simulink model "Quintic_Controller_max_distance"  (R2021a)
settings: Solver=VariableStepAuto  StartTime=0.0  StopTime=1.5  FixedStep=0.00005  MaxStep=.01  RelTol=1e-4  AbsTol=1e-4
values from neighbouring files (symbols this model uses):
  Angle_noise = 0.000001    (= 1e-06)    [Parameters.m]
  Current_noise = 0.000001    (= 1e-06)    [Parameters.m]
  F_sampling = 128    [Parameters.m]
  J_load = J_arm + (J_ball + m_ball*r_arm^2) + J_rotor    (= 0.00716067135)    [Parameters.m]
  J_rotor = 0.0000795    (= 7.95e-05)    [Parameters.m]
  kd_q = 400    [Parameters.m]
  ki_c = 100    [Parameters.m]
  ki_q = 0.01    [Parameters.m]
  ki_s = 4    [Parameters.m]
  km = kt/sqrt(Rm)    [Parameters.m]
  kp_c = 23    [Parameters.m]
  kp_q = 10    [Parameters.m]
  kp_s = 10    [Parameters.m]
  n = 3.75    [Parameters.m]
  nu = 0.85    [Parameters.m]
  Velocity_noise = 0.000001    (= 1e-06)    [Parameters.m]
  x0 = -0.45697770542    [Parameters.m]    (also in getBallPos.m)
  y0 = -0.02848783783    [Parameters.m]    (also in getBallPos.m)
undefined symbols (not defined in the file or in its folder): smiData, X, Y, Z
libraries: sm_lib x103, nesl_utility x12, fl_lib x9, simulink x6, ee_lib x4, spsSampleandHoldLib x3, pid_lib x2, sdl_lib x1
(part 3 of 3)

== system Quintic_Controller_max_distance/Motor ==
  ReferenceFrame : sm_lib/Frames and Transforms/Reference Frame
  Solid : sm_lib/Body Elements/File Solid  ExtGeomFileName=Motor_Default_sldprt.STEP  UnitType=FromFile  ExtGeomFileUnits=m  StepReaderType=HEX  ExportConvexHullGeometry=off  InertiaType=Custom  Mass=smiData.Solid(5).mass  MassUnits=kg  CenterOfMass=smiData.Solid(5).CoM  CenterOfMassUnits=mm  MomentsOfInertia=smiData.Solid(5).MoI  MomentsOfInertiaUnits=kg*mm^2  ProductsOfInertia=smiData.Solid(5).PoI  ProductsOfInertiaUnits=kg*mm^2  BasedOnType=DensityFromFile  Density=1000  DensityUnits=kg/m^3  DoExposeReferenceFrame=on  SerializedFrames=<Frames/>  GraphicType=FromGeometry  MarkerShape=Sphere  MarkerSize=10  GraphicVisPropType=SimpleVisualProperties  GraphicDiffuseColor=smiData.Solid(5).color  GraphicSpecularColor=[0.5 0.5 0.5 1.0]  GraphicAmbientColor=[0.15 0.15 0.15 1.0]  GraphicEmissiveColor=[0.0 0.0 0.0 1.0]  GraphicShininess=75  GraphicOpacity=smiData.Solid(5).opacity
  Transform : sm_lib/Frames and Transforms/Rigid Transform  TranslationMethod=Cartesian  TranslationStandardOffset=0  TranslationLengthUnit=mm  TranslationStandardAxis=+Z  TranslationCartesianOffset=smiData.RigidTransform(28).translation  TranslationROffset=0  TranslationROffsetUnits=m  TranslationZOffset=0  TranslationZOffsetUnits=m  TranslationThetaOffset=0  TranslationThetaOffsetUnits=deg  RotationMethod=ArbitraryAxis  RotationAngleUnits=rad  RotationStandardAxis=+Z  RotationAngle=smiData.RigidTransform(28).angle  RotationArbitraryAxis=smiData.RigidTransform(28).axis  FollAlignAxisA=+X  BaseAlignAxisA=+Y  FollAlignAxisB=+Y  BaseAlignAxisB=+Z  RotationSequenceAxes=FollowerAxes  RotationSequence=XYX  RotationSequenceAngles=[0 0 0]  RotationSequenceAnglesUnits=deg  RotationMatrix=[1 0 0; 0 1 0; 0 0 1]
  Transform1 : sm_lib/Frames and Transforms/Rigid Transform  TranslationMethod=Cartesian  TranslationStandardOffset=0  TranslationLengthUnit=mm  TranslationStandardAxis=+Z  TranslationCartesianOffset=smiData.RigidTransform(45).translation  TranslationROffset=0  TranslationROffsetUnits=m  TranslationZOffset=0  TranslationZOffsetUnits=m  TranslationThetaOffset=0  TranslationThetaOffsetUnits=deg  RotationMethod=ArbitraryAxis  RotationAngleUnits=rad  RotationStandardAxis=+Z  RotationAngle=smiData.RigidTransform(45).angle  RotationArbitraryAxis=smiData.RigidTransform(45).axis  FollAlignAxisA=+X  BaseAlignAxisA=+Y  FollAlignAxisB=+Y  BaseAlignAxisB=+Z  RotationSequenceAxes=FollowerAxes  RotationSequence=XYX  RotationSequenceAngles=[0 0 0]  RotationSequenceAnglesUnits=deg  RotationMatrix=[1 0 0; 0 1 0; 0 0 1]
  F : PMIOPort  Side=Left
  F1 : PMIOPort  Port=2  Side=Right
  connections:
  ReferenceFrame/RConn1 -- Solid/RConn1 -- Transform/LConn1 -- Transform1/LConn1
  Transform/RConn1 -- F/RConn1
  Transform1/RConn1 -- F1/RConn1

== system Quintic_Controller_max_distance/Motor Mount ==
  ReferenceFrame : sm_lib/Frames and Transforms/Reference Frame
  Solid : sm_lib/Body Elements/File Solid  ExtGeomFileName=8982K141_Multipurpose 6061 Aluminum 90 Degree Angle_8982K141_sldprt.STEP  UnitType=FromFile  ExtGeomFileUnits=m  StepReaderType=HEX  ExportConvexHullGeometry=off  InertiaType=Custom  Mass=smiData.Solid(4).mass  MassUnits=kg  CenterOfMass=smiData.Solid(4).CoM  CenterOfMassUnits=in  MomentsOfInertia=smiData.Solid(4).MoI  MomentsOfInertiaUnits=kg*in^2  ProductsOfInertia=smiData.Solid(4).PoI  ProductsOfInertiaUnits=kg*in^2  BasedOnType=DensityFromFile  Density=1000  DensityUnits=kg/m^3  DoExposeReferenceFrame=on  SerializedFrames=<Frames/>  GraphicType=FromGeometry  MarkerShape=Sphere  MarkerSize=10  GraphicVisPropType=SimpleVisualProperties  GraphicDiffuseColor=smiData.Solid(4).color  GraphicSpecularColor=[0.5 0.5 0.5 1.0]  GraphicAmbientColor=[0.15 0.15 0.15 1.0]  GraphicEmissiveColor=[0.0 0.0 0.0 1.0]  GraphicShininess=75  GraphicOpacity=smiData.Solid(4).opacity
  Transform : sm_lib/Frames and Transforms/Rigid Transform  TranslationMethod=Cartesian  TranslationStandardOffset=0  TranslationLengthUnit=mm  TranslationStandardAxis=+Z  TranslationCartesianOffset=smiData.RigidTransform(26).translation  TranslationROffset=0  TranslationROffsetUnits=m  TranslationZOffset=0  TranslationZOffsetUnits=m  TranslationThetaOffset=0  TranslationThetaOffsetUnits=deg  RotationMethod=ArbitraryAxis  RotationAngleUnits=rad  RotationStandardAxis=+Z  RotationAngle=smiData.RigidTransform(26).angle  RotationArbitraryAxis=smiData.RigidTransform(26).axis  FollAlignAxisA=+X  BaseAlignAxisA=+Y  FollAlignAxisB=+Y  BaseAlignAxisB=+Z  RotationSequenceAxes=FollowerAxes  RotationSequence=XYX  RotationSequenceAngles=[0 0 0]  RotationSequenceAnglesUnits=deg  RotationMatrix=[1 0 0; 0 1 0; 0 0 1]
  Transform1 : sm_lib/Frames and Transforms/Rigid Transform  TranslationMethod=Cartesian  TranslationStandardOffset=0  TranslationLengthUnit=mm  TranslationStandardAxis=+Z  TranslationCartesianOffset=smiData.RigidTransform(27).translation  TranslationROffset=0  TranslationROffsetUnits=m  TranslationZOffset=0  TranslationZOffsetUnits=m  TranslationThetaOffset=0  TranslationThetaOffsetUnits=deg  RotationMethod=ArbitraryAxis  RotationAngleUnits=rad  RotationStandardAxis=+Z  RotationAngle=smiData.RigidTransform(27).angle  RotationArbitraryAxis=smiData.RigidTransform(27).axis  FollAlignAxisA=+X  BaseAlignAxisA=+Y  FollAlignAxisB=+Y  BaseAlignAxisB=+Z  RotationSequenceAxes=FollowerAxes  RotationSequence=XYX  RotationSequenceAngles=[0 0 0]  RotationSequenceAnglesUnits=deg  RotationMatrix=[1 0 0; 0 1 0; 0 0 1]
  Transform2 : sm_lib/Frames and Transforms/Rigid Transform  TranslationMethod=Cartesian  TranslationStandardOffset=0  TranslationLengthUnit=mm  TranslationStandardAxis=+Z  TranslationCartesianOffset=smiData.RigidTransform(44).translation  TranslationROffset=0  TranslationROffsetUnits=m  TranslationZOffset=0  TranslationZOffsetUnits=m  TranslationThetaOffset=0  TranslationThetaOffsetUnits=deg  RotationMethod=ArbitraryAxis  RotationAngleUnits=rad  RotationStandardAxis=+Z  RotationAngle=smiData.RigidTransform(44).angle  RotationArbitraryAxis=smiData.RigidTransform(44).axis  FollAlignAxisA=+X  BaseAlignAxisA=+Y  FollAlignAxisB=+Y  BaseAlignAxisB=+Z  RotationSequenceAxes=FollowerAxes  RotationSequence=XYX  RotationSequenceAngles=[0 0 0]  RotationSequenceAnglesUnits=deg  RotationMatrix=[1 0 0; 0 1 0; 0 0 1]
  F1 : PMIOPort  Side=Left
  F2 : PMIOPort  Port=2  Side=Left
  F : PMIOPort  Port=3  Side=Left
  connections:
  ReferenceFrame/RConn1 -- Solid/RConn1 -- Transform/LConn1 -- Transform1/LConn1 -- Transform2/LConn1
  Transform/RConn1 -- F/RConn1
  Transform1/RConn1 -- F1/RConn1
  Transform2/RConn1 -- F2/RConn1

== system Quintic_Controller_max_distance/Output Gear ==
  ReferenceFrame : sm_lib/Frames and Transforms/Reference Frame
  Solid : sm_lib/Body Elements/File Solid  ExtGeomFileName=2664N150_METAL GEAR - 20 DEGREE PRESSURE ANGLE_2664N15_sldprt.STEP  UnitType=FromFile  ExtGeomFileUnits=m  StepReaderType=HEX  ExportConvexHullGeometry=off  InertiaType=Custom  Mass=smiData.Solid(7).mass  MassUnits=kg  CenterOfMass=smiData.Solid(7).CoM  CenterOfMassUnits=in  MomentsOfInertia=smiData.Solid(7).MoI  MomentsOfInertiaUnits=kg*in^2  ProductsOfInertia=smiData.Solid(7).PoI  ProductsOfInertiaUnits=kg*in^2  BasedOnType=DensityFromFile  Density=1000  DensityUnits=kg/m^3  DoExposeReferenceFrame=on  SerializedFrames=<Frames/>  GraphicType=FromGeometry  MarkerShape=Sphere  MarkerSize=10  GraphicVisPropType=SimpleVisualProperties  GraphicDiffuseColor=smiData.Solid(7).color  GraphicSpecularColor=[0.5 0.5 0.5 1.0]  GraphicAmbientColor=[0.15 0.15 0.15 1.0]  GraphicEmissiveColor=[0.0 0.0 0.0 1.0]  GraphicShininess=75  GraphicOpacity=smiData.Solid(7).opacity
  Transform : sm_lib/Frames and Transforms/Rigid Transform  TranslationMethod=Cartesian  TranslationStandardOffset=0  TranslationLengthUnit=mm  TranslationStandardAxis=+Z  TranslationCartesianOffset=smiData.RigidTransform(40).translation  TranslationROffset=0  TranslationROffsetUnits=m  TranslationZOffset=0  TranslationZOffsetUnits=m  TranslationThetaOffset=0  TranslationThetaOffsetUnits=deg  RotationMethod=ArbitraryAxis  RotationAngleUnits=rad  RotationStandardAxis=+Z  RotationAngle=smiData.RigidTransform(40).angle  RotationArbitraryAxis=smiData.RigidTransform(40).axis  FollAlignAxisA=+X  BaseAlignAxisA=+Y  FollAlignAxisB=+Y  BaseAlignAxisB=+Z  RotationSequenceAxes=FollowerAxes  RotationSequence=XYX  RotationSequenceAngles=[0 0 0]  RotationSequenceAnglesUnits=deg  RotationMatrix=[1 0 0; 0 1 0; 0 0 1]
  Transform1 : sm_lib/Frames and Transforms/Rigid Transform  TranslationMethod=Cartesian  TranslationStandardOffset=0  TranslationLengthUnit=mm  TranslationStandardAxis=+Z  TranslationCartesianOffset=smiData.RigidTransform(41).translation  TranslationROffset=0  TranslationROffsetUnits=m  TranslationZOffset=0  TranslationZOffsetUnits=m  TranslationThetaOffset=0  TranslationThetaOffsetUnits=deg  RotationMethod=ArbitraryAxis  RotationAngleUnits=rad  RotationStandardAxis=+Z  RotationAngle=smiData.RigidTransform(41).angle  RotationArbitraryAxis=smiData.RigidTransform(41).axis  FollAlignAxisA=+X  BaseAlignAxisA=+Y  FollAlignAxisB=+Y  BaseAlignAxisB=+Z  RotationSequenceAxes=FollowerAxes  RotationSequence=XYX  RotationSequenceAngles=[0 0 0]  RotationSequenceAnglesUnits=deg  RotationMatrix=[1 0 0; 0 1 0; 0 0 1]
  F : PMIOPort  Side=Left
  F1 : PMIOPort  Port=2  Side=Right
  connections:
  ReferenceFrame/RConn1 -- Solid/RConn1 -- Transform/LConn1 -- Transform1/LConn1
  Transform/RConn1 -- F/RConn1
  Transform1/RConn1 -- F1/RConn1

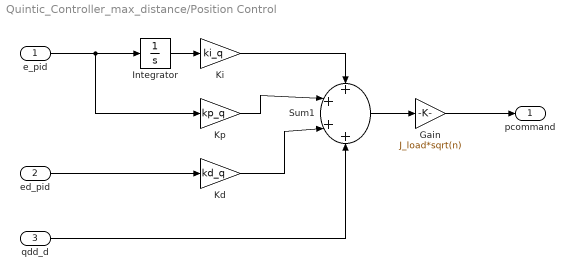
== system Quintic_Controller_max_distance/Position Control ==
  e_pid : Inport
  ed_pid : Inport  Port=2
  qdd_d : Inport  Port=3
  Gain : Gain  Gain=J_load*sqrt(n)
  Integrator : Integrator
  Kd : Gain  Gain=kd_q
  Ki : Gain  Gain=ki_q
  Kp : Gain  Gain=kp_q
  Sum1 : Sum  Inputs=++++
  pcommand : Outport
  wires:
  e_pid/1 -> Integrator/1, Kp/1
  ed_pid/1 -> Kd/1
  Integrator/1 -> Ki/1
  Kp/1 -> Sum1/2
  Sum1/1 -> Gain/1
  Ki/1 -> Sum1/1
  Kd/1 -> Sum1/3
  qdd_d/1 -> Sum1/4
  Gain/1 -> pcommand/1

== system Quintic_Controller_max_distance/Power Sens ==
  Integrator : Integrator
  PS-Simulink Converter8 : nesl_utility/PS-Simulink Converter  PhysicalDomain=network_engine_domain  SubClassName=ps_output  LeftPortType=input  RightPortType=output  PseudoPeriodic=off  Frequencies=[]  Unit=inherit  AffineConversion=off
      settings: SourceProductBaseCode=PW,SS
  Power : Scope
  Power Sensor : ee_lib/Sensors & Transducers/Power Sensor  measurement_type=1  averaging_period=1e-4 s
      settings: SourceProductBaseCode=PS
  To Workspace : ToWorkspace  VariableName=total_power  SaveFormat=Timeseries  SampleTime=-1
  Source : PMIOPort  Side=Left
  + : PMIOPort  Port=2  Side=Left
  GND : PMIOPort  Port=3  Side=Left
  wires:
  PS-Simulink Converter8/1 -> Integrator/1
  Integrator/1 -> To Workspace/1, Power/1
  connections:
  Power Sensor/LConn3 -- GND/RConn1
  Power Sensor/RConn1 -- PS-Simulink Converter8/LConn1
  Power Sensor/LConn2 -- +/RConn1
  Power Sensor/LConn1 -- Source/RConn1

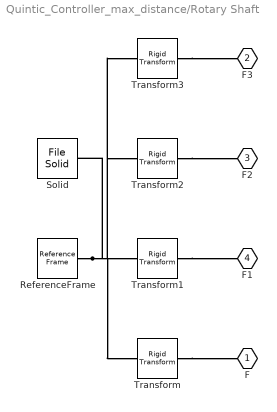
== system Quintic_Controller_max_distance/Rotary Shaft ==
  ReferenceFrame : sm_lib/Frames and Transforms/Reference Frame
  Solid : sm_lib/Body Elements/File Solid  ExtGeomFileName=1439K411_1045 Carbon Steel Keyed Rotary Shaft_1439K411_sldprt.STEP  UnitType=FromFile  ExtGeomFileUnits=m  StepReaderType=HEX  ExportConvexHullGeometry=off  InertiaType=Custom  Mass=smiData.Solid(10).mass  MassUnits=kg  CenterOfMass=smiData.Solid(10).CoM  CenterOfMassUnits=mm  MomentsOfInertia=smiData.Solid(10).MoI  MomentsOfInertiaUnits=kg*mm^2  ProductsOfInertia=smiData.Solid(10).PoI  ProductsOfInertiaUnits=kg*mm^2  BasedOnType=DensityFromFile  Density=1000  DensityUnits=kg/m^3  DoExposeReferenceFrame=on  SerializedFrames=<Frames/>  GraphicType=FromGeometry  MarkerShape=Sphere  MarkerSize=10  GraphicVisPropType=SimpleVisualProperties  GraphicDiffuseColor=smiData.Solid(10).color  GraphicSpecularColor=[0.5 0.5 0.5 1.0]  GraphicAmbientColor=[0.15 0.15 0.15 1.0]  GraphicEmissiveColor=[0.0 0.0 0.0 1.0]  GraphicShininess=75  GraphicOpacity=smiData.Solid(10).opacity
  Transform : sm_lib/Frames and Transforms/Rigid Transform  TranslationMethod=Cartesian  TranslationStandardOffset=0  TranslationLengthUnit=mm  TranslationStandardAxis=+Z  TranslationCartesianOffset=smiData.RigidTransform(24).translation  TranslationROffset=0  TranslationROffsetUnits=m  TranslationZOffset=0  TranslationZOffsetUnits=m  TranslationThetaOffset=0  TranslationThetaOffsetUnits=deg  RotationMethod=ArbitraryAxis  RotationAngleUnits=rad  RotationStandardAxis=+Z  RotationAngle=smiData.RigidTransform(24).angle  RotationArbitraryAxis=smiData.RigidTransform(24).axis  FollAlignAxisA=+X  BaseAlignAxisA=+Y  FollAlignAxisB=+Y  BaseAlignAxisB=+Z  RotationSequenceAxes=FollowerAxes  RotationSequence=XYX  RotationSequenceAngles=[0 0 0]  RotationSequenceAnglesUnits=deg  RotationMatrix=[1 0 0; 0 1 0; 0 0 1]
  Transform1 : sm_lib/Frames and Transforms/Rigid Transform  TranslationMethod=Cartesian  TranslationStandardOffset=0  TranslationLengthUnit=mm  TranslationStandardAxis=+Z  TranslationCartesianOffset=smiData.RigidTransform(29).translation  TranslationROffset=0  TranslationROffsetUnits=m  TranslationZOffset=0  TranslationZOffsetUnits=m  TranslationThetaOffset=0  TranslationThetaOffsetUnits=deg  RotationMethod=ArbitraryAxis  RotationAngleUnits=rad  RotationStandardAxis=+Z  RotationAngle=smiData.RigidTransform(29).angle  RotationArbitraryAxis=smiData.RigidTransform(29).axis  FollAlignAxisA=+X  BaseAlignAxisA=+Y  FollAlignAxisB=+Y  BaseAlignAxisB=+Z  RotationSequenceAxes=FollowerAxes  RotationSequence=XYX  RotationSequenceAngles=[0 0 0]  RotationSequenceAnglesUnits=deg  RotationMatrix=[1 0 0; 0 1 0; 0 0 1]
  Transform2 : sm_lib/Frames and Transforms/Rigid Transform  TranslationMethod=Cartesian  TranslationStandardOffset=0  TranslationLengthUnit=mm  TranslationStandardAxis=+Z  TranslationCartesianOffset=smiData.RigidTransform(37).translation  TranslationROffset=0  TranslationROffsetUnits=m  TranslationZOffset=0  TranslationZOffsetUnits=m  TranslationThetaOffset=0  TranslationThetaOffsetUnits=deg  RotationMethod=ArbitraryAxis  RotationAngleUnits=rad  RotationStandardAxis=+Z  RotationAngle=smiData.RigidTransform(37).angle  RotationArbitraryAxis=smiData.RigidTransform(37).axis  FollAlignAxisA=+X  BaseAlignAxisA=+Y  FollAlignAxisB=+Y  BaseAlignAxisB=+Z  RotationSequenceAxes=FollowerAxes  RotationSequence=XYX  RotationSequenceAngles=[0 0 0]  RotationSequenceAnglesUnits=deg  RotationMatrix=[1 0 0; 0 1 0; 0 0 1]
  Transform3 : sm_lib/Frames and Transforms/Rigid Transform  TranslationMethod=Cartesian  TranslationStandardOffset=0  TranslationLengthUnit=mm  TranslationStandardAxis=+Z  TranslationCartesianOffset=smiData.RigidTransform(39).translation  TranslationROffset=0  TranslationROffsetUnits=m  TranslationZOffset=0  TranslationZOffsetUnits=m  TranslationThetaOffset=0  TranslationThetaOffsetUnits=deg  RotationMethod=ArbitraryAxis  RotationAngleUnits=rad  RotationStandardAxis=+Z  RotationAngle=smiData.RigidTransform(39).angle  RotationArbitraryAxis=smiData.RigidTransform(39).axis  FollAlignAxisA=+X  BaseAlignAxisA=+Y  FollAlignAxisB=+Y  BaseAlignAxisB=+Z  RotationSequenceAxes=FollowerAxes  RotationSequence=XYX  RotationSequenceAngles=[0 0 0]  RotationSequenceAnglesUnits=deg  RotationMatrix=[1 0 0; 0 1 0; 0 0 1]
  F : PMIOPort  Side=Left
  F3 : PMIOPort  Port=2  Side=Right
  F2 : PMIOPort  Port=3  Side=Right
  F1 : PMIOPort  Port=4  Side=Right
  connections:
  ReferenceFrame/RConn1 -- Solid/RConn1 -- Transform/LConn1 -- Transform1/LConn1 -- Transform2/LConn1 -- Transform3/LConn1
  Transform/RConn1 -- F/RConn1
  Transform1/RConn1 -- F1/RConn1
  Transform2/RConn1 -- F2/RConn1
  Transform3/RConn1 -- F3/RConn1

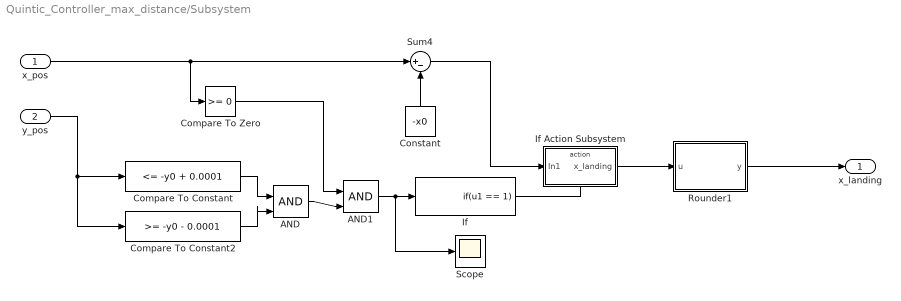
== system Quintic_Controller_max_distance/Subsystem ==
  x_pos : Inport
  y_pos : Inport  Port=2
  AND : Logic  IconShape=distinctive  AllPortsSameDT=off  OutDataTypeStr=boolean
  AND1 : Logic  IconShape=distinctive  AllPortsSameDT=off  OutDataTypeStr=boolean
  Compare To Constant : simulink/Logic and Bit Operations/Compare To Constant  relop=<=  const=-y0 + 0.0001  OutDataTypeStr=boolean
  Compare To Constant2 : simulink/Logic and Bit Operations/Compare To Constant  relop=>=  const=-y0 - 0.0001  OutDataTypeStr=boolean
  Compare To Zero : simulink/Logic and Bit Operations/Compare To Zero  relop=>=  OutDataTypeStr=boolean
  Constant : Constant  Value=-x0
  If : If  IfExpression=u1 == 1  ShowElse=off
  If Action Subsystem : Subsystem  TreatAsAtomicUnit=on
  Rounder1 : MATLAB Function  TreatAsAtomicUnit=on
  Scope : Scope
  Sum4 : Sum  Inputs=|+-
  x_landing : Outport
  wires:
  AND/1 -> AND1/2
  Compare To Constant2/1 -> AND/2
  y_pos/1 -> Compare To Constant2/1, Compare To Constant/1
  If/1 -> If Action Subsystem/Action
  Compare To Constant/1 -> AND/1
  Compare To Zero/1 -> AND1/1
  AND1/1 -> Scope/1, If/1
  Sum4/1 -> If Action Subsystem/1(In1)
  x_pos/1 -> Sum4/1, Compare To Zero/1
  Constant/1 -> Sum4/2
  If Action Subsystem/1(x_landing) -> Rounder1/1(u)
  Rounder1/1(y) -> x_landing/1

== system Quintic_Controller_max_distance/Velocity Sample//Noise Selector ==
  In1 : Inport
  Noise3 : Subsystem
  Sample3 : Subsystem  Commented=through
  Switch1 : Switch  Criteria=u2 > Threshold
  Switch2 : Switch  Criteria=u2 > Threshold
  Velocity Noise : Constant  Value=0
  Velocity Sample : Constant  Value=0
  Out1 : Outport
  wires:
  Switch1/1 -> Switch2/3, Sample3/1(In1)
  Sample3/1("   ") -> Switch2/1
  Velocity Noise/1 -> Switch1/2
  Switch2/1 -> Out1/1
  In1/1 -> Noise3/1(In1), Switch1/3
  Noise3/1(Out1) -> Switch1/1
  Velocity Sample/1 -> Switch2/2

== system Quintic_Controller_max_distance/Angle Sample//Noise Selector1/Noise3 ==
  In1 : Inport
  Band-Limited White Noise : simulink/Sources/Band-Limited White Noise  Cov=[Angle_noise]  Ts=0.001  seed=[23341]
  Sum3 : Sum  Inputs=|++
  Out1 : Outport
  wires:
  Band-Limited White Noise/1 -> Sum3/1
  In1/1 -> Sum3/2
  Sum3/1 -> Out1/1

== system Quintic_Controller_max_distance/Angle Sample//Noise Selector1/Sample3 ==
  In1 : Inport
  Pulse Generator : DiscretePulseGenerator  PulseType=Time based  Period=1/F_sampling
  Sample and Hold : spsSampleandHoldLib/Sample and Hold  ic=0  Ts=0
      settings: SourceProductBaseCode=PS
  "   " : Outport
  wires:
  Pulse Generator/1 -> Sample and Hold/2
  Sample and Hold/1 -> "   "/1
  In1/1 -> Sample and Hold/1

== system Quintic_Controller_max_distance/Current Sample//Noise Selector/Noise3 ==
  In1 : Inport
  Band-Limited White Noise : simulink/Sources/Band-Limited White Noise  Cov=[Current_noise]  Ts=0.001  seed=[23341]
  Sum3 : Sum  Inputs=|++
  Out1 : Outport
  wires:
  Band-Limited White Noise/1 -> Sum3/1
  In1/1 -> Sum3/2
  Sum3/1 -> Out1/1

== system Quintic_Controller_max_distance/Current Sample//Noise Selector/Sample3 ==
  In1 : Inport
  Pulse Generator : DiscretePulseGenerator  PulseType=Time based  Period=1/F_sampling
  Sample and Hold : spsSampleandHoldLib/Sample and Hold  ic=0  Ts=0
      settings: SourceProductBaseCode=PS
  "   " : Outport
  wires:
  Pulse Generator/1 -> Sample and Hold/2
  Sample and Hold/1 -> "   "/1
  In1/1 -> Sample and Hold/1

== system Quintic_Controller_max_distance/Subsystem/If Action Subsystem ==
  In1 : Inport
  Action Port : ActionPort  ActionPortLabel=if(u1 == 1)
  x_landing : Outport
  wires:
  In1/1 -> x_landing/1

== system Quintic_Controller_max_distance/Velocity Sample//Noise Selector/Noise3 ==
  In1 : Inport
  Band-Limited White Noise : simulink/Sources/Band-Limited White Noise  Cov=[Velocity_noise]  Ts=0.001  seed=[23341]
  Sum3 : Sum  Inputs=|++
  Out1 : Outport
  wires:
  Band-Limited White Noise/1 -> Sum3/1
  In1/1 -> Sum3/2
  Sum3/1 -> Out1/1

== system Quintic_Controller_max_distance/Velocity Sample//Noise Selector/Sample3 ==
  In1 : Inport
  Pulse Generator : DiscretePulseGenerator  PulseType=Time based  Period=1/F_sampling
  Sample and Hold : spsSampleandHoldLib/Sample and Hold  ic=0  Ts=0
      settings: SourceProductBaseCode=PS
  "   " : Outport
  wires:
  Pulse Generator/1 -> Sample and Hold/2
  Sample and Hold/1 -> "   "/1
  In1/1 -> Sample and Hold/1

== matlab function Quintic_Controller_max_distance/Trajectory Calculator ==
  data: T_ramp output; W_cruise output; T_fin output; T_ret output; a_ret output; q_ret output; W_cruise input; test_num input
function [T_ramp, W_cruise, T_fin, T_ret, a_ret, q_ret]= fcn(W_cruise, test_num)

a_ret = -100;

if test_num == 1
    q_ret = 25/36*pi;
    T_ramp = 0.08;
    T_ret = (q_ret - 0.5*W_cruise*T_ramp)/W_cruise + T_ramp;
    T_fin = 0.2;
elseif test_num == 2
    q_ret = 4/9*pi;
    T_ramp = 0.065;
    T_ret = (q_ret - 0.5*W_cruise*T_ramp)/W_cruise + T_ramp;
    T_fin = 0.15;
else
    q_ret = 0;
    T_ramp = 0;
    T_ret = 0;
    T_fin = 0;
end

== matlab function Quintic_Controller_max_distance/MATLAB Function ==
  data: command input; tau output; pcommand input; theta input; t input; T_ramp input; W_cruise input; T_fin input; T_ret input; a_ret input; q_ret input; omega input; e_pid output; ed_pid output; q_d output; qd_d output; qdd_d output
 function [tau, e_pid, ed_pid, q_d, qd_d, qdd_d] = fcn(command, pcommand, theta, t, T_ramp, W_cruise, T_fin, T_ret, a_ret, q_ret, omega)
 
 if (t <= T_ramp)
     q_d = 0.5 * W_cruise * t^2/T_ramp;
     qd_d = W_cruise * t/T_ramp;
     qdd_d = W_cruise/T_ramp;
     e_pid = qd_d - omega;
     tau = command;
     q_0=[];
     q_1=[];
     q_2=[];
     q_3=[];
     ed_pid = 0;
     
 elseif (t > T_ramp & t < T_ret)
     q_d = 0.5 * W_cruise * T_ramp + W_cruise * (t-T_ramp);
     qd_d = W_cruise;
     qdd_d = 0;
     e_pid = qd_d - omega;
     tau = command;
     q_0=[];
     q_1=[];
     q_2=[];
     q_3=[];
     ed_pid = 0;
     
 elseif (t >= T_ret & t < T_fin)
     Del = T_fin - T_ret;
     q_2 = a_ret*0.5;
     q_1 = W_cruise;
     q_0 = q_ret;
     ii = inv([Del^3 Del^4 Del^5; 3*Del^2 4*Del^3 5*Del^4; 6*Del 12*Del^2 20*Del^3])*[(-q_0 - q_1*Del - q_2*Del^2); (-q_1 - 2*q_2*Del); -2*q_2];
     
     q_3=ii(1); q_4=ii(2); q_5=ii(3);
     Del_T= t- T_ret;
     
     q_d = q_0 + q_1*Del_T + q_2*Del_T^2 + q_3*Del_T^3 + q_4*Del_T^4 + q_5*Del_T^5;
     qd_d = q_1 + 2*q_2*Del_T + 3*q_3*Del_T^2 + 4*q_4*Del_T^3 + 5*q_5*Del_T^4;
     qdd_d = 2*q_2 + 6*q_3*Del_T + 12*q_4*Del_T^2 + 20*q_5*Del_T^3;
     e_pid = q_d - theta;
     ed_pid = qd_d - omega;
     tau = pcommand;
    
 else 
     q_d = 0;
     qd_d = 0;
     qdd_d = 0;
     e_pid = q_d - theta;
     ed_pid = qd_d - omega;
     tau = pcommand;
 end

== matlab function Quintic_Controller_max_distance/Subsystem/Rounder1 ==
  data: u input; y output
function y = fcn(u)

f = 10.^2;
y = round(f*u)/f;
